simulink model "sim_IL_H2DF_2024a"  (R2024a)
settings: Solver=FixedStepAuto  StartTime=0.0  StopTime=4899  FixedStep=1  RelTol=1e-3  EnableMultiTasking=on
model workspace (MAT data in the model file):
  enable_IMEP_noise = 100
  enable_IMEP_offset = 1
values from neighbouring files (symbols this model uses):
  IL = struct()    [init_simulink_IL_H2DF.m]
undefined symbols (not defined in the file or in its folder): C2C_NMPC, cost_length, horizon_length, y_ref_buf
libraries: dspswit3 x4, deeplib x1
(part 2 of 2)

== system sim_IL_H2DF_2024a/reference/reference_dynamic_random_steps/reference_dynamic_smoothened_random/Enabled Subsystem ==
  Enable : EnablePort
  Uniform Random Number : UniformRandomNumber  Minimum=400000  Maximum=800000  Seed=5
  Uniform Random Number1 : UniformRandomNumber  Minimum=15  Maximum=150  VectorParams1D=off
  num : Outport
  freq : Outport  Port=2
  wires:
  Uniform Random Number1/1 -> freq/1
  Uniform Random Number/1 -> num/1

== system sim_IL_H2DF_2024a/reference/reference_dynamic_smoothened_random_fast_steps/reference_dynamic_smoothened_random/Enabled Subsystem ==
  Enable : EnablePort
  Uniform Random Number : UniformRandomNumber  Minimum=400000  Maximum=800000  Seed=1
  Uniform Random Number1 : UniformRandomNumber  Minimum=15  Maximum=150  VectorParams1D=off
  num : Outport
  freq : Outport  Port=2
  wires:
  Uniform Random Number1/1 -> freq/1
  Uniform Random Number/1 -> num/1

== system sim_IL_H2DF_2024a/reference/reference_dynamic_smoothened_random_slow_steps/reference_dynamic_smoothened_random/Enabled Subsystem ==
  Enable : EnablePort
  Uniform Random Number : UniformRandomNumber  Minimum=400000  Maximum=800000  Seed=1
  Uniform Random Number1 : UniformRandomNumber  Minimum=15  Maximum=150  VectorParams1D=off
  num : Outport
  freq : Outport  Port=2
  wires:
  Uniform Random Number1/1 -> freq/1
  Uniform Random Number/1 -> num/1

== system sim_IL_H2DF_2024a/dynamics/Plant From MPC/Hardcoded/dyn_H2DF/dyn_H2DF ==
  controls : Inport
  last_outputs : Inport  Port=2
  last_LSTM_states : Inport  Port=3
  Terminator : Terminator
  dyn_H2DF : MATLAB Function  TreatAsAtomicUnit=on
  outputs : Outport
  wires:
  last_LSTM_states/1 -> dyn_H2DF/1(last_LSTM_states)
  dyn_H2DF/2(LSTM_states) -> Terminator/1
  controls/1 -> dyn_H2DF/2(controls)
  dyn_H2DF/1(outputs) -> outputs/1
  last_outputs/1 -> dyn_H2DF/3(last_outputs)

== system sim_IL_H2DF_2024a/dynamics/Plant From MPC/Hardcoded/dyn_H2DF_state_augmentation/dyn_H2DF_state_augmentation ==
  last_LSTM_states : Inport
  controls : Inport  Port=2
  last_outputs : Inport  Port=3
  dyn_H2DF_state_augmentation : MATLAB Function  TreatAsAtomicUnit=on
  LSTM_states : Outport
  wires:
  dyn_H2DF_state_augmentation/1(LSTM_states) -> LSTM_states/1
  last_outputs/1 -> dyn_H2DF_state_augmentation/3(last_outputs)
  last_LSTM_states/1 -> dyn_H2DF_state_augmentation/1(last_LSTM_states)
  controls/1 -> dyn_H2DF_state_augmentation/2(controls)

== matlab function sim_IL_H2DF_2024a/dynamics/Plant From MPC/Hardcoded/dyn_H2DF/dyn_H2DF/dyn_H2DF ==
  data: last_LSTM_states input; controls input; last_outputs input; outputs output; H2DF_Par parameter; LSTM_states output
function [outputs, LSTM_states] = dyn_H2DF(last_LSTM_states, controls, last_outputs, H2DF_Par)

[outputs, LSTM_states] = dyn_H2DF_GRU(last_LSTM_states, [controls; last_outputs(1)], H2DF_Par);

== matlab function sim_IL_H2DF_2024a/reference/reference_dynamic_smoothened/reference_dynamic_smoothened/ref_func ==
  data: ref_norm input; y_ref output size=horizon_length * cost_length; init_index input size=1; y_ref_buf parameter; cost_length parameter size=1; horizon_length parameter size=1
function y_ref = ref_func(ref_norm, init_index, y_ref_buf, cost_length, horizon_length)
% more init in callbacks

% init output
y_ref = zeros(cost_length*horizon_length, 1);

if init_index == 4899
    y_ref_buf(:, 1) = ref_norm(:, init_index);
    y_ref_buf(:, 2) = ref_norm(:, init_index+1);
    y_ref_buf(:, 3) = ref_norm(:, init_index+1);
elseif init_index == 4900
    y_ref_buf(:, 1) = ref_norm(:, init_index);
    y_ref_buf(:, 2) = ref_norm(:, init_index);
    y_ref_buf(:, 3) = ref_norm(:, init_index);
else
    y_ref_buf(:, 1) = ref_norm(:, init_index);
    y_ref_buf(:, 2) = ref_norm(:, init_index+1);
    y_ref_buf(:, 3) = ref_norm(:, init_index+2); 
end

y_ref(1:cost_length) = y_ref_buf(:,1);
y_ref( (cost_length+1) : (cost_length * 2) ) = y_ref_buf(:,2);
y_ref( ((cost_length*2)+1) : (cost_length * 3) ) = y_ref_buf(:,3);

== matlab function sim_IL_H2DF_2024a/reference/reference_static/ref_func ==
  data: ref_norm input; y_ref output; init_index input
function y_ref = ref_func(ref_norm, init_index)

y_ref = ref_norm(:, init_index);

== matlab function sim_IL_H2DF_2024a/dynamics/Plant From MPC/Hardcoded/dyn_H2DF_state_augmentation/dyn_H2DF_state_augmentation/dyn_H2DF_state_augmentation ==
  data: last_LSTM_states input; LSTM_states output; controls input; last_outputs input; H2DF_Par parameter
function LSTM_states = dyn_H2DF_state_augmentation(last_LSTM_states, controls, last_outputs, H2DF_Par)

LSTM_states = dyn_H2DF_state_augmentation_GRU(last_LSTM_states,[controls; last_outputs(1)], H2DF_Par);

== matlab function sim_IL_H2DF_2024a/reference/reference_dynamic_constant/reference_dynamic_constant/ref_func ==
  data: ref_norm input; y_ref output size=horizon_length * cost_length; init_index input size=1; y_ref_buf parameter; cost_length parameter size=1; horizon_length parameter size=1
function y_ref = ref_func(ref_norm, init_index, y_ref_buf, cost_length, horizon_length)
% more init in callbacks

% init output
y_ref = zeros(cost_length*horizon_length, 1);

if init_index == 4899
    y_ref_buf(:, 1) = ref_norm(:, init_index);
    y_ref_buf(:, 2) = ref_norm(:, init_index+1);
    y_ref_buf(:, 3) = ref_norm(:, init_index+1);
elseif init_index == 4900
    y_ref_buf(:, 1) = ref_norm(:, init_index);
    y_ref_buf(:, 2) = ref_norm(:, init_index);
    y_ref_buf(:, 3) = ref_norm(:, init_index);
else
    y_ref_buf(:, 1) = ref_norm(:, init_index);
    y_ref_buf(:, 2) = ref_norm(:, init_index+1);
    y_ref_buf(:, 3) = ref_norm(:, init_index+2); 
end

y_ref(1:cost_length) = y_ref_buf(:,1);
y_ref( (cost_length+1) : (cost_length * 2) ) = y_ref_buf(:,2);
y_ref( ((cost_length*2)+1) : (cost_length * 3) ) = y_ref_buf(:,3);

== matlab function sim_IL_H2DF_2024a/reference/reference_dynamic_smoothened_random_slow_steps/reference_dynamic_smoothened_random/ref_func ==
  data: ref_norm input; y_ref output size=horizon_length * cost_length; init_index input size=1; y_ref_buf parameter; cost_length parameter size=1; horizon_length parameter size=1
function y_ref = ref_func(ref_norm, init_index, y_ref_buf, cost_length, horizon_length)
% more init in callbacks

% init output
y_ref = zeros(cost_length*horizon_length, 1);

if init_index == 4899
    y_ref_buf(:, 1) = ref_norm(:, init_index);
    y_ref_buf(:, 2) = ref_norm(:, init_index+1);
    y_ref_buf(:, 3) = ref_norm(:, init_index+1);
elseif init_index == 4900
    y_ref_buf(:, 1) = ref_norm(:, init_index);
    y_ref_buf(:, 2) = ref_norm(:, init_index);
    y_ref_buf(:, 3) = ref_norm(:, init_index);
else
    y_ref_buf(:, 1) = ref_norm(:, init_index);
    y_ref_buf(:, 2) = ref_norm(:, init_index+1);
    y_ref_buf(:, 3) = ref_norm(:, init_index+2); 
end

y_ref(1:cost_length) = y_ref_buf(:,1);
y_ref( (cost_length+1) : (cost_length * 2) ) = y_ref_buf(:,2);
y_ref( ((cost_length*2)+1) : (cost_length * 3) ) = y_ref_buf(:,3);

== matlab function sim_IL_H2DF_2024a/reference/reference_dynamic_random_steps/reference_dynamic_smoothened_random/ref_func ==
  data: ref_norm input; y_ref output size=horizon_length * cost_length; init_index input size=1; y_ref_buf parameter; cost_length parameter size=1; horizon_length parameter size=1
function y_ref = ref_func(ref_norm, init_index, y_ref_buf, cost_length, horizon_length)
% more init in callbacks

% init output
y_ref = zeros(cost_length*horizon_length, 1);

if init_index == 4899
    y_ref_buf(:, 1) = ref_norm(:, init_index);
    y_ref_buf(:, 2) = ref_norm(:, init_index+1);
    y_ref_buf(:, 3) = ref_norm(:, init_index+1);
elseif init_index == 4900
    y_ref_buf(:, 1) = ref_norm(:, init_index);
    y_ref_buf(:, 2) = ref_norm(:, init_index);
    y_ref_buf(:, 3) = ref_norm(:, init_index);
else
    y_ref_buf(:, 1) = ref_norm(:, init_index);
    y_ref_buf(:, 2) = ref_norm(:, init_index+1);
    y_ref_buf(:, 3) = ref_norm(:, init_index+2); 
end

y_ref(1:cost_length) = y_ref_buf(:,1);
y_ref( (cost_length+1) : (cost_length * 2) ) = y_ref_buf(:,2);
y_ref( ((cost_length*2)+1) : (cost_length * 3) ) = y_ref_buf(:,3);

== matlab function sim_IL_H2DF_2024a/reference/reference_dynamic_smoothened_random_fast_steps/reference_dynamic_smoothened_random/ref_func ==
  data: ref_norm input; y_ref output size=horizon_length * cost_length; init_index input size=1; y_ref_buf parameter; cost_length parameter size=1; horizon_length parameter size=1
function y_ref = ref_func(ref_norm, init_index, y_ref_buf, cost_length, horizon_length)
% more init in callbacks

% init output
y_ref = zeros(cost_length*horizon_length, 1);

if init_index == 4899
    y_ref_buf(:, 1) = ref_norm(:, init_index);
    y_ref_buf(:, 2) = ref_norm(:, init_index+1);
    y_ref_buf(:, 3) = ref_norm(:, init_index+1);
elseif init_index == 4900
    y_ref_buf(:, 1) = ref_norm(:, init_index);
    y_ref_buf(:, 2) = ref_norm(:, init_index);
    y_ref_buf(:, 3) = ref_norm(:, init_index);
else
    y_ref_buf(:, 1) = ref_norm(:, init_index);
    y_ref_buf(:, 2) = ref_norm(:, init_index+1);
    y_ref_buf(:, 3) = ref_norm(:, init_index+2); 
end

y_ref(1:cost_length) = y_ref_buf(:,1);
y_ref( (cost_length+1) : (cost_length * 2) ) = y_ref_buf(:,2);
y_ref( ((cost_length*2)+1) : (cost_length * 3) ) = y_ref_buf(:,3);

== matlab function sim_IL_H2DF_2024a/reference/reference_dynamic/reference_dynamic/ref_func ==
  data: ref_norm input; y_ref output size=horizon_length * cost_length; init_index input size=1; y_ref_buf parameter; cost_length parameter size=1; horizon_length parameter size=1
function y_ref = ref_func(ref_norm, init_index, y_ref_buf, cost_length, horizon_length)
% more init in callbacks

% init output
y_ref = zeros(cost_length*horizon_length, 1);

if init_index == 4899
    y_ref_buf(:, 1) = ref_norm(:, init_index);
    y_ref_buf(:, 2) = ref_norm(:, init_index+1);
    y_ref_buf(:, 3) = ref_norm(:, init_index+1);
elseif init_index == 4900
    y_ref_buf(:, 1) = ref_norm(:, init_index);
    y_ref_buf(:, 2) = ref_norm(:, init_index);
    y_ref_buf(:, 3) = ref_norm(:, init_index);
else
    y_ref_buf(:, 1) = ref_norm(:, init_index);
    y_ref_buf(:, 2) = ref_norm(:, init_index+1);
    y_ref_buf(:, 3) = ref_norm(:, init_index+2); 
end

y_ref(1:cost_length) = y_ref_buf(:,1);
y_ref( (cost_length+1) : (cost_length * 2) ) = y_ref_buf(:,2);
y_ref( ((cost_length*2)+1) : (cost_length * 3) ) = y_ref_buf(:,3);
